simulink model "PlantTest"  (R2018b)
settings: Solver=VariableStepAuto  StartTime=0.0  StopTime=10.0  RelTol=1e-3
undefined symbols (not defined in the file): a, b, c, cyl_init_length, d, diffz, init_beta1, omegaR, steer
libraries: simulink x2
settings Model: Creator=ogihara  LastModifiedBy=ogihara

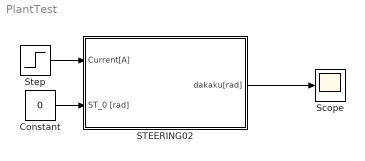
== system PlantTest ==
  Constant : Constant  Value=0
  STEERING02 : Subsystem  Description=|
      | Current: STバルブスプール電流の (右出
      | ST_0: ステア角 初期値
      mask Display:
      | patch([0 0 1 1], [0.98 0.96 0.96 0.98], [1 0.5 0])
      | patch([0 0 1 1], [0.02 0.04 0.04 0.02], [1 0.5 0])
  Scope : Scope
  Step : Step  SampleTime=0
  wires:
  Constant/1 -> STEERING02/2(ST_0 [rad])
  STEERING02/1(dakaku[rad]) -> Scope/1
  Step/1 -> STEERING02/1(Current[A])

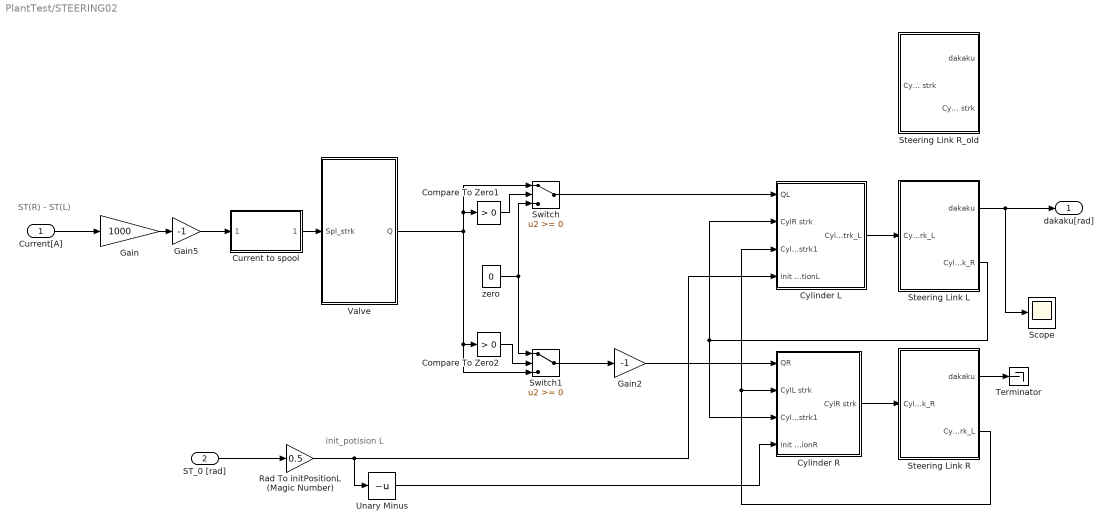
== system PlantTest/STEERING02 ==
  note: init_potision L
  note: ST(R) - ST(L)
  Current[A] : Inport
  ST_0 [rad] : Inport  Port=2
  " Valve" : Subsystem
  Compare To Zero1 : simulink/Logic and Bit Operations/Compare To Zero  relop=>  OutDataTypeStr=boolean
  Compare To Zero2 : simulink/Logic and Bit Operations/Compare To Zero  relop=>  OutDataTypeStr=boolean
  Current to spool : Subsystem
  Cylinder L : Subsystem
  Cylinder R : Subsystem
  Gain : Gain  Gain=1000
  Gain2 : Gain  Gain=-1
  Gain5 : Gain  Gain=-1
  Rad To initPositionL (Magic Number) : Gain  Gain=0.5
  Scope : Scope
  Steering Link L : Subsystem
  Steering Link R : Subsystem
  Steering Link R_old : Subsystem
  Switch : Switch
  Switch1 : Switch
  Terminator : Terminator
  Unary Minus : UnaryMinus
  zero : Constant  Value=0
  dakaku[rad] : Outport
  wires:
  Current to spool/1(Spl_strk) -> " Valve"/1(Spl_strk)
  Current[A]/1 -> Gain/1
  Steering Link L/2(Cyl_strk_R) -> Cylinder L/2(CylR strk), Cylinder R/3(CylR strk1)
  Gain5/1 -> Current to spool/1(Current)
  Steering Link R/2(Cyl_strk_L) -> Cylinder L/3(CylL strk1), Cylinder R/2(CylL strk)
  Cylinder L/1(Cyl_strk_L) -> Steering Link L/1(Cyl_strk_L)
  Cylinder R/1(CylR strk) -> Steering Link R/1(Cyl_strk_R)
  Unary Minus/1 -> Cylinder R/4(init positionR)
  Gain2/1 -> Cylinder R/1(QR)
  Switch/1 -> Cylinder L/1(QL)
  " Valve"/1(Q) -> Switch/1, Compare To Zero1/1, Switch1/3, Compare To Zero2/1
  Switch1/1 -> Gain2/1
  zero/1 -> Switch/3, Switch1/1
  Steering Link R/1(dakaku) -> Terminator/1
  Gain/1 -> Gain5/1
  ST_0 [rad]/1 -> Rad To initPositionL (Magic Number)/1
  Rad To initPositionL (Magic Number)/1 -> Cylinder L/4(init positionL), Unary Minus/1
  Steering Link L/1(dakaku) -> dakaku[rad]/1, Scope/1
  Compare To Zero1/1 -> Switch/2
  Compare To Zero2/1 -> Switch1/2

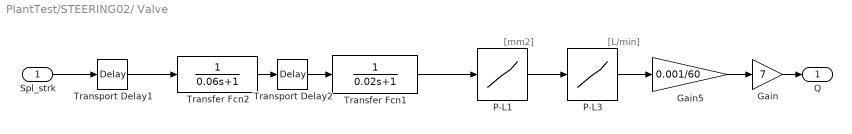
== system PlantTest/STEERING02/ Valve ==
  note: [mm2]
  note: [L/min]
  Spl_strk : Inport
  Gain : Gain  Gain=7
  Gain5 : Gain  Gain=0.001/60  SaturateOnIntegerOverflow=on  OutDataTypeStr=Inherit: Same as input  ParamDataTypeStr=Inherit: Same as input
  P-L1 : Lookup  InputValues=[-7 -6 -5.5 -5 -4 -3 -2 0 2 3 4 5 5.5 6 7]  Table=[-35 -15 -9 -7.4 -4.2 -1.4 0 0 0 1.4 4.2 7.4 9 15 35]  SaturateOnIntegerOverflow=on
  P-L3 : Lookup  InputValues=[-35 -15 -7.4 -5.8 -4.2 -2.8 -1.4 -0.7 -0.28 0 0.28 0.7 1.4 2.8 4.2 5.8 7.4 15 35]  Table=[-35.5 -15.3 -9.7 -7.4 -5.4 -3.6 -2.15 -1.1 -0.6 0 0.6 1.1 2.15 3.6 5.4 7.4 9.7 15.3 35.5]  SaturateOnIntegerOverflow=on
  Transfer Fcn1 : TransferFcn  Denominator=[0.02 1]
  Transfer Fcn2 : TransferFcn  Denominator=[0.06 1]
  Transport Delay1 : TransportDelay  DelayTime=0.1
  Transport Delay2 : TransportDelay  DelayTime=0.05
  Q : Outport
  wires:
  Spl_strk/1 -> Transport Delay1/1
  P-L1/1 -> P-L3/1
  Gain/1 -> Q/1
  Gain5/1 -> Gain/1
  P-L3/1 -> Gain5/1
  Transport Delay1/1 -> Transfer Fcn2/1
  Transport Delay2/1 -> Transfer Fcn1/1
  Transfer Fcn1/1 -> P-L1/1
  Transfer Fcn2/1 -> Transport Delay2/1

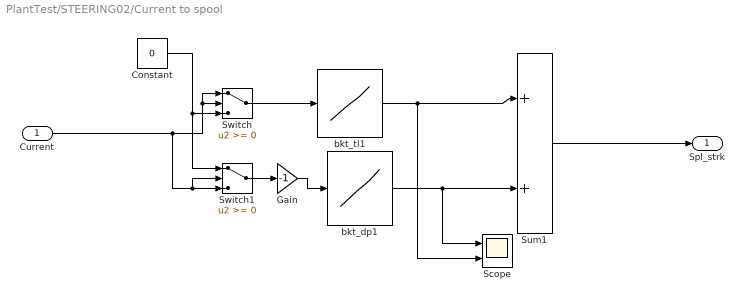
== system PlantTest/STEERING02/Current to spool ==
  Current : Inport
  Constant : Constant  Value=0
  Gain : Gain  Gain=-1
  Scope : Scope  NumInputPorts=2
  Sum1 : Sum  SaturateOnIntegerOverflow=on
  Switch : Switch
  Switch1 : Switch
  bkt_dp1 : Lookup  InputValues=[0 400 450 500 550 600 650 1000]  Table=[0 -2 -3 -4 -5 -6 -7 -7]  SaturateOnIntegerOverflow=on
  bkt_tl1 : Lookup  InputValues=[0 400 450 500 550 600 650 1000]  Table=[0 2 3 4 5 6 7 7]  SaturateOnIntegerOverflow=on
  Spl_strk : Outport
  wires:
  bkt_tl1/1 -> Sum1/1, Scope/2
  Current/1 -> Switch/2, Switch/1, Switch1/3, Switch1/2
  Switch/1 -> bkt_tl1/1
  Constant/1 -> Switch/3, Switch1/1
  Switch1/1 -> Gain/1
  Gain/1 -> bkt_dp1/1
  bkt_dp1/1 -> Sum1/2, Scope/1
  Sum1/1 -> Spl_strk/1

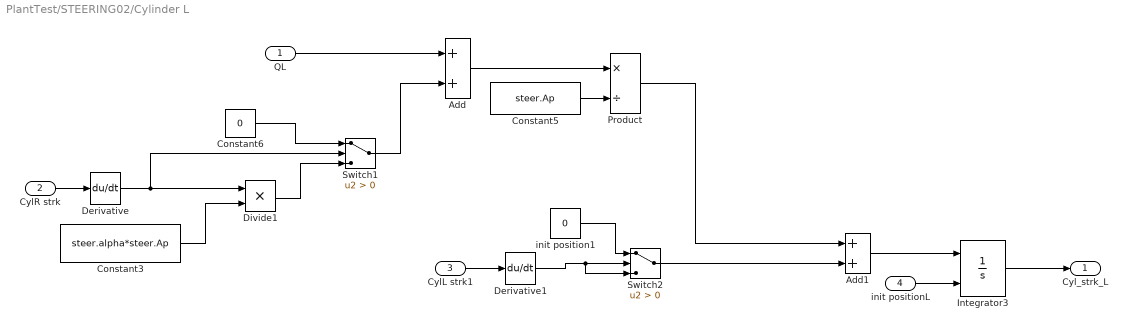
== system PlantTest/STEERING02/Cylinder L ==
  QL : Inport
  CylR strk : Inport  Port=2
  CylL strk1 : Inport  Port=3
  init positionL : Inport  Port=4
  Add : Sum
  Add1 : Sum
  Constant3 : Constant  Value=steer.alpha*steer.Ap
  Constant5 : Constant  Value=steer.Ap
  Constant6 : Constant  Value=0
  Derivative : Derivative
  Derivative1 : Derivative
  Divide1 : Product  Inputs=**
  Integrator3 : Integrator  InitialConditionSource=external  LimitOutput=on  UpperSaturationLimit=steer.xpmax  LowerSaturationLimit=steer.xpmin
  Product : Product  Inputs=*/  RndMeth=Zero
  Switch1 : Switch  Criteria=u2 > Threshold
  Switch2 : Switch  Criteria=u2 > Threshold
  init position1 : Constant  Value=0
  Cyl_strk_L : Outport
  wires:
  CylR strk/1 -> Derivative/1
  QL/1 -> Add/1
  Add/1 -> Product/1
  Constant3/1 -> Divide1/2
  Divide1/1 -> Switch1/3
  Derivative/1 -> Divide1/1, Switch1/2
  Switch1/1 -> Add/2
  Constant6/1 -> Switch1/1
  Integrator3/1 -> Cyl_strk_L/1
  Constant5/1 -> Product/2
  Product/1 -> Add1/1
  init positionL/1 -> Integrator3/2
  CylL strk1/1 -> Derivative1/1
  Derivative1/1 -> Switch2/2, Switch2/3
  Add1/1 -> Integrator3/1
  Switch2/1 -> Add1/2
  init position1/1 -> Switch2/1

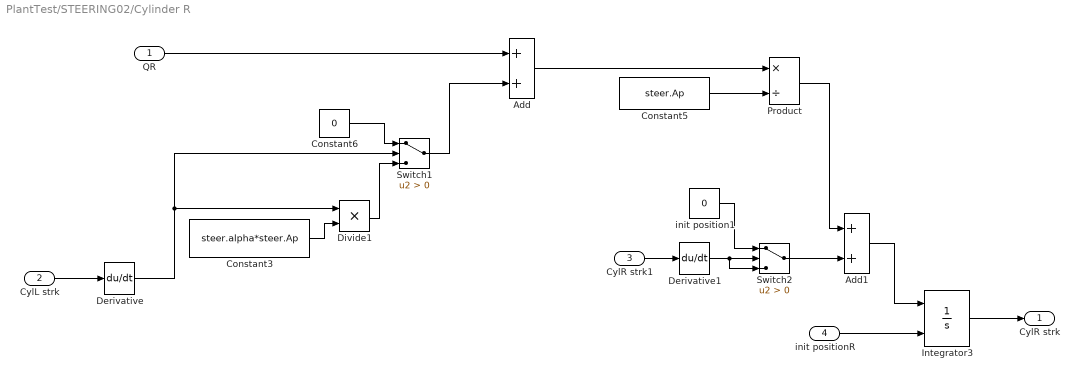
== system PlantTest/STEERING02/Cylinder R ==
  QR : Inport
  CylL strk : Inport  Port=2
  CylR strk1 : Inport  Port=3
  init positionR : Inport  Port=4
  Add : Sum
  Add1 : Sum
  Constant3 : Constant  Value=steer.alpha*steer.Ap
  Constant5 : Constant  Value=steer.Ap
  Constant6 : Constant  Value=0
  Derivative : Derivative
  Derivative1 : Derivative
  Divide1 : Product  Inputs=**
  Integrator3 : Integrator  InitialConditionSource=external  LimitOutput=on  UpperSaturationLimit=steer.xpmax  LowerSaturationLimit=steer.xpmin
  Product : Product  Inputs=*/  RndMeth=Zero
  Switch1 : Switch  Criteria=u2 > Threshold
  Switch2 : Switch  Criteria=u2 > Threshold
  init position1 : Constant  Value=0
  CylR strk : Outport
  wires:
  init positionR/1 -> Integrator3/2
  Product/1 -> Add1/1
  Constant5/1 -> Product/2
  Integrator3/1 -> CylR strk/1
  Constant6/1 -> Switch1/1
  Switch1/1 -> Add/2
  Derivative/1 -> Switch1/2, Divide1/1
  Divide1/1 -> Switch1/3
  Constant3/1 -> Divide1/2
  Add/1 -> Product/1
  QR/1 -> Add/1
  CylL strk/1 -> Derivative/1
  Derivative1/1 -> Switch2/2, Switch2/3
  Add1/1 -> Integrator3/1
  Switch2/1 -> Add1/2
  CylR strk1/1 -> Derivative1/1
  init position1/1 -> Switch2/1

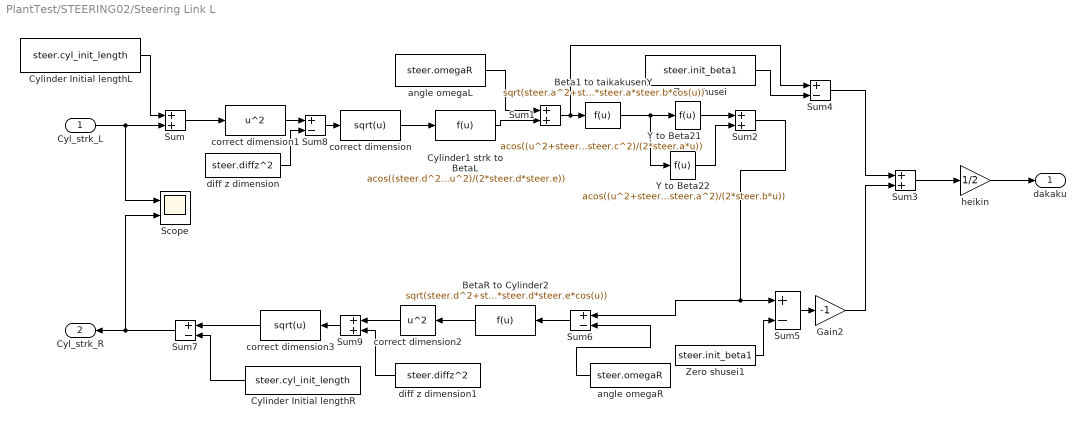
== system PlantTest/STEERING02/Steering Link L ==
  Cyl_strk_L : Inport
  Beta1 to taikakusenY : Fcn  Expr=sqrt(steer.a^2+steer.b^2-2*steer.a*steer.b*cos(u))
  BetaR to Cylinder2 : Fcn  Expr=sqrt(steer.d^2+steer.e^2-2*steer.d*steer.e*cos(u))
  Cylinder Initial lengthL : Constant  Value=steer.cyl_init_length
  Cylinder Initial lengthR : Constant  Value=steer.cyl_init_length
  Cylinder1 strk to BetaL : Fcn  Expr=acos((steer.d^2+steer.e^2-u^2)/(2*steer.d*steer.e))
  Gain2 : Gain  Gain=-1
  Scope : Scope  NumInputPorts=2
  Sum{,1..3,9} (5 alike) : Sum
  Sum{4..8} (5 alike) : Sum  Inputs=+-
  Y to Beta21 : Fcn  Expr=acos((u^2+steer.a^2-steer.c^2)/(2*steer.a*u))
  Y to Beta22 : Fcn  Expr=acos((u^2+steer.b^2-steer.a^2)/(2*steer.b*u))
  Zero shusei : Constant  Value=steer.init_beta1
  Zero shusei1 : Constant  Value=steer.init_beta1
  angle omegaL : Constant  Value=steer.omegaR
  angle omegaR : Constant  Value=steer.omegaR
  correct dimension : Fcn  Expr=sqrt(u)
  correct dimension1 : Fcn  Expr=u^2
  correct dimension2 : Fcn  Expr=u^2
  correct dimension3 : Fcn  Expr=sqrt(u)
  diff z dimension : Constant  Value=steer.diffz^2
  diff z dimension1 : Constant  Value=steer.diffz^2
  heikin : Gain  Gain=1/2
  dakaku : Outport
  Cyl_strk_R : Outport  Port=2
  wires:
  Sum1/1 -> Beta1 to taikakusenY/1, Sum4/1
  Sum3/1 -> heikin/1
  Cylinder1 strk to BetaL/1 -> Sum1/2
  Sum4/1 -> Sum3/1
  Zero shusei/1 -> Sum4/2
  Zero shusei1/1 -> Sum5/2
  Sum5/1 -> Gain2/1
  Gain2/1 -> Sum3/2
  Cyl_strk_L/1 -> Sum/2, Scope/1
  heikin/1 -> dakaku/1
  angle omegaR/1 -> Sum6/2
  Sum6/1 -> BetaR to Cylinder2/1
  Cylinder Initial lengthR/1 -> Sum7/2
  BetaR to Cylinder2/1 -> correct dimension2/1
  Sum7/1 -> Cyl_strk_R/1, Scope/2
  angle omegaL/1 -> Sum1/1
  Cylinder Initial lengthL/1 -> Sum/1
  Sum/1 -> correct dimension1/1
  diff z dimension/1 -> Sum8/2
  correct dimension1/1 -> Sum8/1
  Sum8/1 -> correct dimension/1
  correct dimension/1 -> Cylinder1 strk to BetaL/1
  correct dimension2/1 -> Sum9/1
  Sum9/1 -> correct dimension3/1
  diff z dimension1/1 -> Sum9/2
  correct dimension3/1 -> Sum7/1
  Sum2/1 -> Sum6/1, Sum5/1
  Beta1 to taikakusenY/1 -> Y to Beta21/1, Y to Beta22/1
  Y to Beta21/1 -> Sum2/1
  Y to Beta22/1 -> Sum2/2

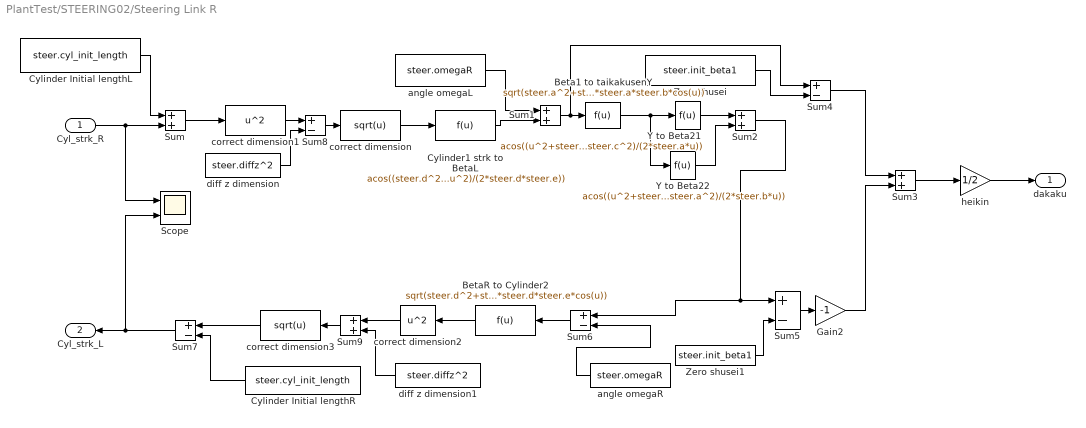
== system PlantTest/STEERING02/Steering Link R ==
  Cyl_strk_R : Inport
  Beta1 to taikakusenY : Fcn  Expr=sqrt(steer.a^2+steer.b^2-2*steer.a*steer.b*cos(u))
  BetaR to Cylinder2 : Fcn  Expr=sqrt(steer.d^2+steer.e^2-2*steer.d*steer.e*cos(u))
  Cylinder Initial lengthL : Constant  Value=steer.cyl_init_length
  Cylinder Initial lengthR : Constant  Value=steer.cyl_init_length
  Cylinder1 strk to BetaL : Fcn  Expr=acos((steer.d^2+steer.e^2-u^2)/(2*steer.d*steer.e))
  Gain2 : Gain  Gain=-1
  Scope : Scope  NumInputPorts=2
  Sum{,1..3,9} (5 alike) : Sum
  Sum{4..8} (5 alike) : Sum  Inputs=+-
  Y to Beta21 : Fcn  Expr=acos((u^2+steer.a^2-steer.c^2)/(2*steer.a*u))
  Y to Beta22 : Fcn  Expr=acos((u^2+steer.b^2-steer.a^2)/(2*steer.b*u))
  Zero shusei : Constant  Value=steer.init_beta1
  Zero shusei1 : Constant  Value=steer.init_beta1
  angle omegaL : Constant  Value=steer.omegaR
  angle omegaR : Constant  Value=steer.omegaR
  correct dimension : Fcn  Expr=sqrt(u)
  correct dimension1 : Fcn  Expr=u^2
  correct dimension2 : Fcn  Expr=u^2
  correct dimension3 : Fcn  Expr=sqrt(u)
  diff z dimension : Constant  Value=steer.diffz^2
  diff z dimension1 : Constant  Value=steer.diffz^2
  heikin : Gain  Gain=1/2
  dakaku : Outport
  Cyl_strk_L : Outport  Port=2
  wires:
  Sum1/1 -> Beta1 to taikakusenY/1, Sum4/1
  Sum3/1 -> heikin/1
  Cylinder1 strk to BetaL/1 -> Sum1/2
  Sum4/1 -> Sum3/1
  Zero shusei/1 -> Sum4/2
  Zero shusei1/1 -> Sum5/2
  Sum5/1 -> Gain2/1
  Gain2/1 -> Sum3/2
  Cyl_strk_R/1 -> Sum/2, Scope/1
  heikin/1 -> dakaku/1
  angle omegaR/1 -> Sum6/2
  Sum6/1 -> BetaR to Cylinder2/1
  Cylinder Initial lengthR/1 -> Sum7/2
  BetaR to Cylinder2/1 -> correct dimension2/1
  Sum7/1 -> Cyl_strk_L/1, Scope/2
  angle omegaL/1 -> Sum1/1
  Cylinder Initial lengthL/1 -> Sum/1
  Sum/1 -> correct dimension1/1
  diff z dimension/1 -> Sum8/2
  correct dimension1/1 -> Sum8/1
  Sum8/1 -> correct dimension/1
  correct dimension/1 -> Cylinder1 strk to BetaL/1
  correct dimension2/1 -> Sum9/1
  Sum9/1 -> correct dimension3/1
  diff z dimension1/1 -> Sum9/2
  correct dimension3/1 -> Sum7/1
  Sum2/1 -> Sum6/1, Sum5/1
  Beta1 to taikakusenY/1 -> Y to Beta21/1, Y to Beta22/1
  Y to Beta21/1 -> Sum2/1
  Y to Beta22/1 -> Sum2/2

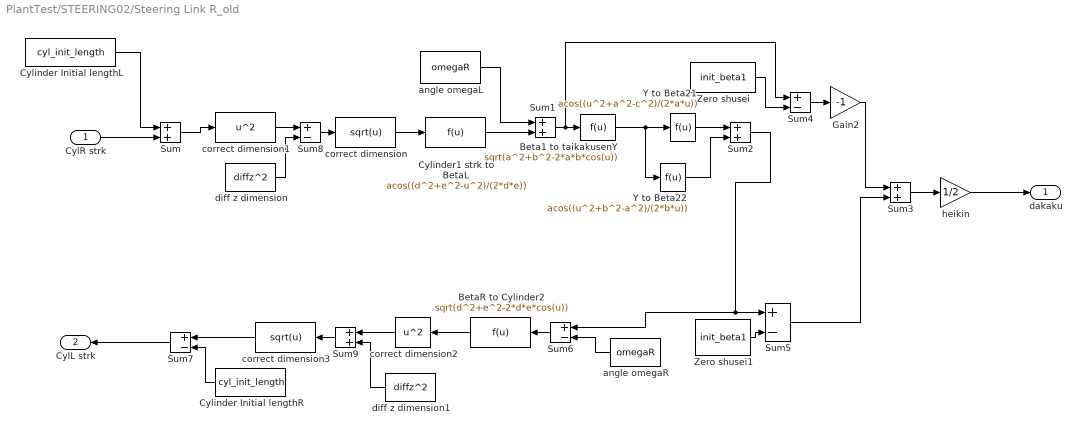
== system PlantTest/STEERING02/Steering Link R_old ==
  CylR strk : Inport
  Beta1 to taikakusenY : Fcn  Expr=sqrt(a^2+b^2-2*a*b*cos(u))
  BetaR to Cylinder2 : Fcn  Expr=sqrt(d^2+e^2-2*d*e*cos(u))
  Cylinder Initial lengthL : Constant  Value=cyl_init_length
  Cylinder Initial lengthR : Constant  Value=cyl_init_length
  Cylinder1 strk to BetaL : Fcn  Expr=acos((d^2+e^2-u^2)/(2*d*e))
  Gain2 : Gain  Gain=-1
  Sum{,1..3,9} (5 alike) : Sum
  Sum{4..8} (5 alike) : Sum  Inputs=+-
  Y to Beta21 : Fcn  Expr=acos((u^2+a^2-c^2)/(2*a*u))
  Y to Beta22 : Fcn  Expr=acos((u^2+b^2-a^2)/(2*b*u))
  Zero shusei : Constant  Value=init_beta1
  Zero shusei1 : Constant  Value=init_beta1
  angle omegaL : Constant  Value=omegaR
  angle omegaR : Constant  Value=omegaR
  correct dimension : Fcn  Expr=sqrt(u)
  correct dimension1 : Fcn  Expr=u^2
  correct dimension2 : Fcn  Expr=u^2
  correct dimension3 : Fcn  Expr=sqrt(u)
  diff z dimension : Constant  Value=diffz^2
  diff z dimension1 : Constant  Value=diffz^2
  heikin : Gain  Gain=1/2
  dakaku : Outport
  CylL strk : Outport  Port=2
  wires:
  Y to Beta22/1 -> Sum2/2
  Y to Beta21/1 -> Sum2/1
  Beta1 to taikakusenY/1 -> Y to Beta22/1, Y to Beta21/1
  Sum2/1 -> Sum5/1, Sum6/1
  correct dimension3/1 -> Sum7/1
  diff z dimension1/1 -> Sum9/2
  Sum9/1 -> correct dimension3/1
  correct dimension2/1 -> Sum9/1
  correct dimension/1 -> Cylinder1 strk to BetaL/1
  Sum8/1 -> correct dimension/1
  correct dimension1/1 -> Sum8/1
  diff z dimension/1 -> Sum8/2
  Sum/1 -> correct dimension1/1
  Cylinder Initial lengthL/1 -> Sum/1
  angle omegaL/1 -> Sum1/1
  Sum7/1 -> CylL strk/1
  BetaR to Cylinder2/1 -> correct dimension2/1
  Cylinder Initial lengthR/1 -> Sum7/2
  Sum6/1 -> BetaR to Cylinder2/1
  angle omegaR/1 -> Sum6/2
  heikin/1 -> dakaku/1
  CylR strk/1 -> Sum/2
  Sum5/1 -> Sum3/2
  Zero shusei1/1 -> Sum5/2
  Zero shusei/1 -> Sum4/2
  Sum4/1 -> Gain2/1
  Cylinder1 strk to BetaL/1 -> Sum1/2
  Sum3/1 -> heikin/1
  Sum1/1 -> Beta1 to taikakusenY/1, Sum4/1
  Gain2/1 -> Sum3/1
